simulink model "Projectile_1D_WithDrag_Soln"  (R2025a)
settings: Solver=VariableStepAuto  StartTime=0.0  StopTime=15  MaxStep=1e-2  RelTol=1e-3
settings Model: Creator=esmithzb  LastModifiedBy=esmithzb

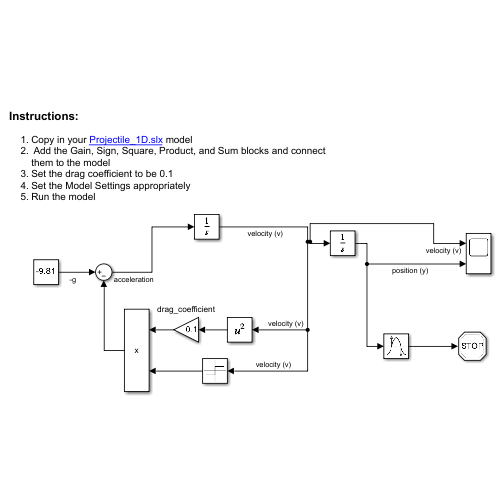
[thumbnail: Simulink's stored preview of the top-level diagram]
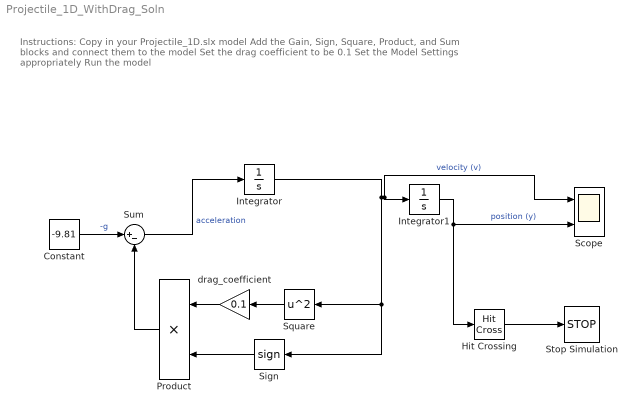
== system Projectile_1D_WithDrag_Soln ==
  note: Instructions:
      |
      | Copy in your Projectile_1D.slx model
      | Add the Gain, Sign, Square, Product, and Sum blocks and connect them to the model
      | Set the drag coefficient to be 0.1
      | Set the Model Settings appropriately
      | Run the model
  Constant : Constant  Value=-9.81
  Hit Crossing : HitCross
  Integrator : Integrator  InitialCondition=50
  Integrator1 : Integrator  InitialCondition=10
  Product : Product
  Scope : Scope  NumInputPorts=2
      settings: ActiveDisplayYMinimum=-60.36250000000237  ActiveDisplayYMaximum=62.262500000000259  YLabel=meters per second
  Sign : Signum
  Square : Math  Operator=square
  Stop Simulation : Stop
  Sum : Sum  Inputs=|+-
  drag_coefficient : Gain  Gain=0.1
  wires:
  Hit Crossing/1 -> Stop Simulation/1
  Integrator/1 -> Square/1, Sign/1, Integrator1/1, Scope/1  "velocity (v)"
  Integrator1/1 -> Hit Crossing/1, Scope/2  "position (y)"
  Square/1 -> drag_coefficient/1
  Sign/1 -> Product/2
  Product/1 -> Sum/2
  Sum/1 -> Integrator/1  "acceleration"
  Constant/1 -> Sum/1  "-g"
  drag_coefficient/1 -> Product/1
